simulink model "Punkt_3"  (R2018b)
settings: Solver=VariableStepAuto  StartTime=0.0  StopTime=2  MaxStep=0.01  RelTol=1e-3
values from neighbouring files (symbols this model uses):
  A = [0 1; 4 0]    [Punkt_1_sylvesler.m]
  A_sh = [Gf zeros(2); zeros(2) A]    [Raschoty.m]
  B = [1; 1]    [Punkt_1_sylvesler.m]
  B_sh = [zeros(2,1); B]    [Raschoty.m]
  C = [3 0]    [Punkt_1_sylvesler.m]
  C_sh = [Hf C]    [Raschoty.m]
  D = 3    [Punkt_1_sylvesler.m]
  Gf = [0 1; -9 0]    [Raschoty.m]
  Hf = [1 0]    [Raschoty.m]
  L_sh = transpose(-Hn_sh * inv(Mn))    [Raschoty.m]
undefined symbols (not defined in the file or in its folder): Kk, Lf_O
settings Model: Creator=kekos  LastModifiedBy=kekos

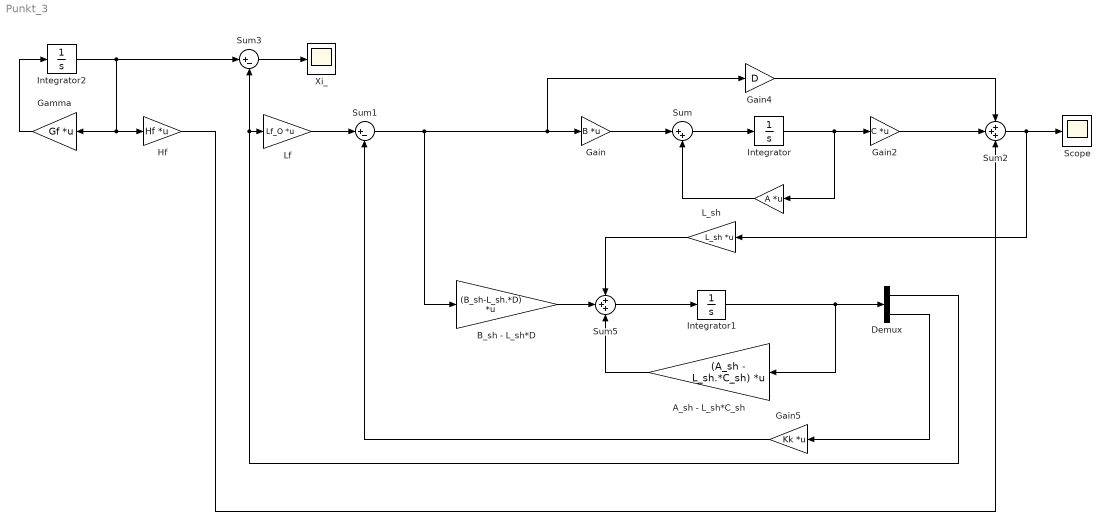
== system Punkt_3 ==
  " " : Gain  Gain=A  Multiplication=Matrix(K*u)
  A_sh - L_sh*C_sh : Gain  Gain=(A_sh - L_sh.*C_sh)  Multiplication=Matrix(K*u)
  B_sh - L_sh*D : Gain  Gain=(B_sh-L_sh.*D)  Multiplication=Matrix(K*u)
  Demux : Demux  Outputs=2
  Gain : Gain  Gain=B  Multiplication=Matrix(K*u)
  Gain2 : Gain  Gain=C  Multiplication=Matrix(K*u)
  Gain4 : Gain  Gain=D
  Gain5 : Gain  Gain=Kk  Multiplication=Matrix(K*u)
  Gamma : Gain  Gain=Gf  Multiplication=Matrix(K*u)
  Hf : Gain  Gain=Hf  Multiplication=Matrix(K*u)
  Integrator : Integrator
  Integrator1 : Integrator  InitialCondition=[1; 0; 1; 1]
  Integrator2 : Integrator  InitialCondition=[-2.91; -19.1]
  L_sh : Gain  Gain=L_sh  Multiplication=Matrix(K*u)
  "Lf " : Gain  Gain=Lf_O  Multiplication=Matrix(K*u)
  Scope : Scope
  Sum : Sum  Inputs=|++
  Sum1 : Sum  Inputs=|+-
  Sum2 : Sum  Inputs=+++
  Sum3 : Sum  Inputs=|+-
  Sum5 : Sum  Inputs=+++
  Xi_ : Scope
  wires:
  Gain4/1 -> Sum2/1
  Gamma/1 -> Integrator2/1
  " "/1 -> Sum/2
  "Lf "/1 -> Sum1/1
  Gain2/1 -> Sum2/2
  Integrator/1 -> Gain2/1, " "/1
  Sum2/1 -> L_sh/1, Scope/1
  Gain5/1 -> Sum1/2
  Sum/1 -> Integrator/1
  Gain/1 -> Sum/1
  Sum1/1 -> B_sh - L_sh*D/1, Gain4/1, Gain/1
  Integrator2/1 -> Sum3/1, Gamma/1, Hf/1
  Hf/1 -> Sum2/3
  Demux/1 -> Sum3/2, "Lf "/1
  Demux/2 -> Gain5/1
  B_sh - L_sh*D/1 -> Sum5/2
  L_sh/1 -> Sum5/1
  A_sh - L_sh*C_sh/1 -> Sum5/3
  Sum5/1 -> Integrator1/1
  Integrator1/1 -> Demux/1, A_sh - L_sh*C_sh/1
  Sum3/1 -> Xi_/1
